simulink model "sensor_codegen_discrete"  (R2022a)
settings: Solver=FixedStepDiscrete  StartTime=0.0  StopTime=12  FixedStep=0.005  RelTol=1e-3
settings Model: Creator=HJL  LastModifiedBy=HJL
settings DataIOCC: SaveOutput=off  SignalLogging=off  DSMLogging=off  SaveTime=off
settings OptimizationCC: ZeroExternalMemoryAtStartup=off  ZeroInternalMemoryAtStartup=off
settings RTWCC: GenCodeOnly=on  TargetLang=C++
settings GRTTargetCC: TargetLangStandard=C++11 (ISO)  MatFileLogging=off  CodeInterfacePackaging=C++ class

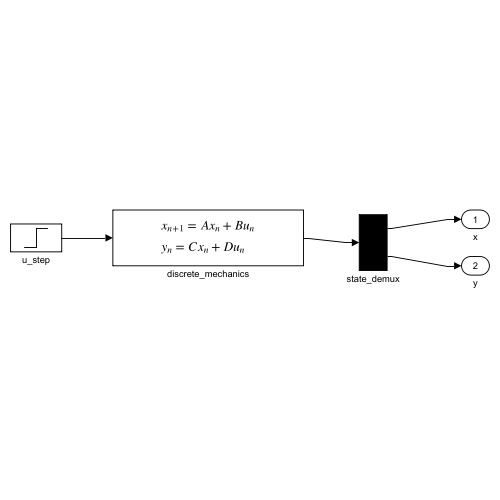
[thumbnail: Simulink's stored preview of the top-level diagram]
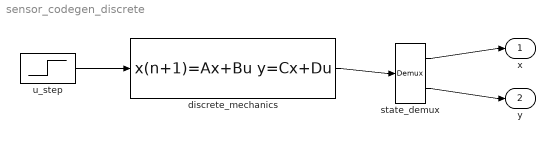
== system sensor_codegen_discrete ==
  discrete_mechanics : DiscreteStateSpace  A=[0.9999850050362352 0.004997475845658773;-0.005996971014790528 0.9989855098671034]  B=[1.249580313731981e-05;0.004997475845658774]  C=[1 0; 0 1]  D=[0; 0]  InitialCondition=[0; 0]  SampleTime=0.005
  state_demux : Demux  Outputs=2
  u_step : Step  SampleTime=0.005
  x : Outport
  y : Outport  Port=2
  wires:
  u_step/1 -> discrete_mechanics/1
  discrete_mechanics/1 -> state_demux/1
  state_demux/1 -> x/1
  state_demux/2 -> y/1
